simulink model "SHA256Simulink"  (R2024a)
settings: Solver=FixedStepAuto  StartTime=0.0  StopTime=0  FixedStep=0.01  RelTol=1e-3
libraries: AVE_Library x1
settings Model: Creator=Scythe  LastModifiedBy=Scythe
settings SolverCC: ConcurrentTasks=on
settings DataIOCC: SaveOutput=off  SignalLogging=off  DSMLogging=off  SaveTime=off  ReturnWorkspaceOutputs=off
settings OptimizationCC: DefaultParameterBehavior=Inlined  ZeroExternalMemoryAtStartup=off  ZeroInternalMemoryAtStartup=off  SimCompilerOptimization=on
settings DebuggingCC: UnconnectedInputMsg=warning  UnconnectedOutputMsg=warning  UnconnectedLineMsg=warning
settings HardwareCC: ProdBitPerLong=64  ProdHWDeviceType=Intel->x86-64 (Linux 64)
settings ModelReferenceCC: EnableRefExpFcnMdlSchedulingChecks=on
settings SFSimCC: SimParseCustomCode=off  SimGenImportedTypeDefs=on  SimTargetLang=C++
settings RTWCC: GenCodeOnly=on  PackageGeneratedCodeAndArtifacts=on  PackageName=PackNGo  RTWVerbose=off  BuildConfiguration=Faster Runs  TargetLang=C++
settings CodeAppCC: ForceParamTrailComments=on  MaxIdLength=128  StateflowObjectComments=on  MATLABSourceComments=on  UseSimReservedNames=on
settings GRTTargetCC: TargetLangStandard=C++11 (ISO)  MatFileLogging=off  CodeInterfacePackaging=C++ class

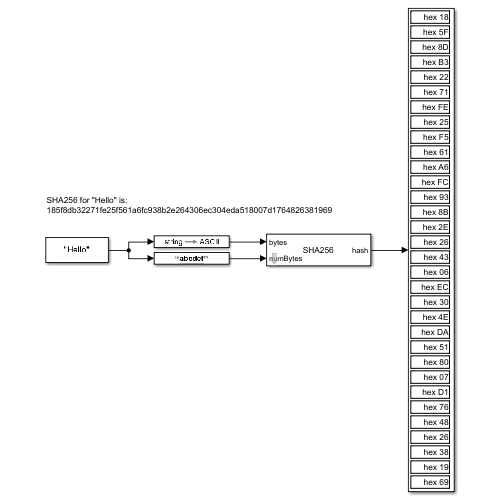
[thumbnail: Simulink's stored preview of the top-level diagram]
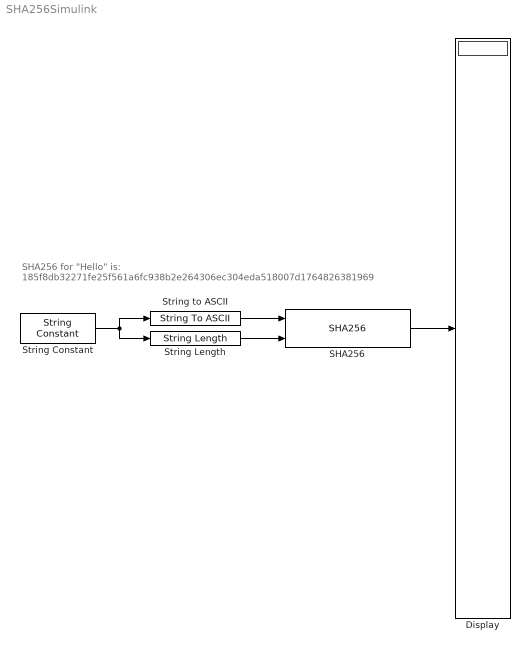
== system SHA256Simulink ==
  note: SHA256 for "Hello" is:
      | 185f8db32271fe25f561a6fc938b2e264306ec304eda518007d1764826381969
  Display : Display
      settings: Format=hex (Stored Integer)
  SHA256 : AVE_Library/Essential/SHA256
      settings: SourceProductName=AVE - Autonomous Vehicle Control Toolbox
  String Constant : StringConstant  String="\"Hello\""
  String Length : StringLength
  String to ASCII : StringToASCII
  wires:
  SHA256/1 -> Display/1
  String Constant/1 -> String to ASCII/1, String Length/1
  String Length/1 -> SHA256/2
  String to ASCII/1 -> SHA256/1
